simulink model "model"  (R2024a)
settings: Solver=FixedStepAuto  StartTime=0.0  StopTime=100  FixedStep=0.01  RelTol=1e-3
undefined symbols (not defined in the file or in its folder): e0_0, e1_0, e2_0, e3_0, q0, Thrust, vec
libraries: sharedtransform x21, sharedutil x4, aerolibsim3d x2, dspsigops x2, shared6dof x1, sim3dlib x1
(part 2 of 2)

== system model/Quadrotor/Forces in Body frame/Thrust in Inertia Frame ==
  DCM_be : Inport
  Thrust : Inport  Port=2
  Mux : Mux  Inputs=3
  Product1 : Product  Multiplication=Matrix(*)  InputSameDT=on  SaturateOnIntegerOverflow=on  OutDataTypeStr=Inherit: Same as first input
  Reshape : Reshape  OutputDimensionality=Column vector (2-D)
  Transpose : Math  Operator=transpose
  x : Constant  Value=0  SampleTime=-1
  y : Constant  Value=0  SampleTime=-1
  U : Outport
  wires:
  Product1/1 -> U/1
  Mux/1 -> Reshape/1
  y/1 -> Mux/2
  x/1 -> Mux/1
  Reshape/1 -> Product1/2
  Thrust/1 -> Mux/3
  DCM_be/1 -> Transpose/1
  Transpose/1 -> Product1/1

== system model/Quadrotor in body/6DOF NED/Angular Velocity Dyanmics ==
  Moments : Inport  OutDataTypeStr=double
  Bus Creator1 : BusCreator  Inputs=3
  Bus Creator2 : BusCreator  Inputs=3
  Centrifugal Moments : Subsystem
  Demux1 : Demux  Outputs=3
  Demux2 : Demux  Outputs=3
  Inertia Matrix : Constant  Value=InertiaMatrix
  Product2 : Product  Inputs=*/  Multiplication=Matrix(*)  SaturateOnIntegerOverflow=on  OutDataTypeStr=Inherit: Same as first input
  Reshape : Reshape
  Reshape1 : Reshape  OutputDimensionality=Row vector (2-D)
  Sum2 : Sum  Inputs=++|  SaturateOnIntegerOverflow=on
  Wdot Integ : Integrator  InitialCondition=OmegaInitialValues  ContinuousStateAttributes={'p', 'q', 'r'}
  W : Outport
  Wdot : Outport  Port=2  OutDataTypeStr=double  Unit=rad/s^2  VectorParamsAs1DForOutWhenUnconnected=off
  wires:
  Bus Creator2/1 -> Wdot/1  "Wdot"
  Demux2/1 -> Bus Creator2/1  "pdot"
  Demux2/3 -> Bus Creator2/3  "rdot"
  Demux2/2 -> Bus Creator2/2  "qdot"
  Reshape/1 -> Wdot Integ/1, Demux2/1
  Sum2/1 -> Reshape1/1
  Bus Creator1/1 -> Centrifugal Moments/1(w), W/1  "W"
  Demux1/2 -> Bus Creator1/2  "q"
  Demux1/3 -> Bus Creator1/3  "r"
  Wdot Integ/1 -> Demux1/1
  Demux1/1 -> Bus Creator1/1  "p"
  Reshape1/1 -> Product2/1
  Moments/1 -> Sum2/1
  Inertia Matrix/1 -> Product2/2
  Centrifugal Moments/1((I * w) x w) -> Sum2/2
  Product2/1 -> Reshape/1

== system model/Quadrotor in body/6DOF NED/Quaternion Dynamics ==
  w : Inport
  Integrating : Subsystem
  Mux : Mux  Inputs=2
  Quat to Euler : Subsystem
  Quaternions to Direction Cosine Matrix : sharedtransform/Quaternions to  Direction Cosine Matrix  aMode=aMode
  q0_dot : Subsystem
  qvec_dot : Subsystem
  DCM_be : Outport  OutDataTypeStr=double  VectorParamsAs1DForOutWhenUnconnected=off
  Quat : Outport  Port=2  OutDataTypeStr=double  VectorParamsAs1DForOutWhenUnconnected=off
  Euler : Outport  Port=3  OutDataTypeStr=double  VectorParamsAs1DForOutWhenUnconnected=off
  wires:
  Quat to Euler/1(euler) -> Euler/1
  Mux/1 -> Integrating/1(qdot)
  w/1 -> q0_dot/1(w), qvec_dot/1(w)
  Quaternions to Direction Cosine Matrix/1 -> DCM_be/1
  q0_dot/1(q0_dot) -> Mux/1
  qvec_dot/1(qvec_dot) -> Mux/2
  Integrating/1(Quat) -> qvec_dot/2(q), q0_dot/2(q), Quat to Euler/1(q), Quaternions to Direction Cosine Matrix/1, Quat/1

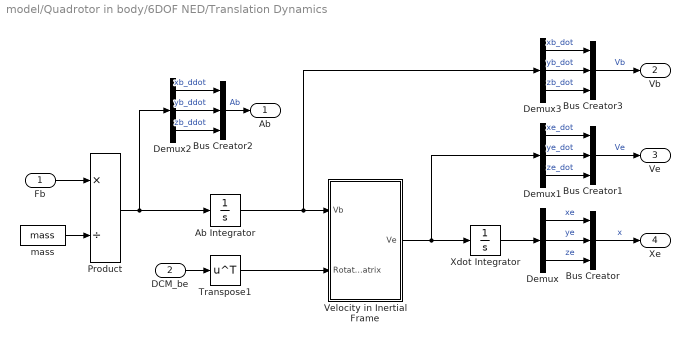
== system model/Quadrotor in body/6DOF NED/Translation Dynamics ==
  Fb : Inport
  DCM_be : Inport  Port=2
  Ab Integrator : Integrator  InitialCondition=VelocityBodyInitialValues  ContinuousStateAttributes={'u', 'v', 'w'}
  Bus Creator{,1..3} (4 alike) : BusCreator  Inputs=3
  Demux{,1..3} (4 alike) : Demux  Outputs=3
  Product : Product  Inputs=*/
  Transpose1 : Math  Operator=transpose  SignedPower=on
  Velocity in Inertial Frame : Subsystem
  Xdot Integrator : Integrator  InitialCondition=PositionReferenceInitialValues  ContinuousStateAttributes={'xr', 'ye', 'ze'}
  mass : Constant  Value=mass
  Ab : Outport  OutDataTypeStr=double  Unit=m/s^2  VectorParamsAs1DForOutWhenUnconnected=off
  Vb : Outport  Port=2  OutDataTypeStr=double  Unit=m/s  VectorParamsAs1DForOutWhenUnconnected=off
  Ve : Outport  Port=3  OutDataTypeStr=double  Unit=m/s  VectorParamsAs1DForOutWhenUnconnected=off
  Xe : Outport  Port=4
  wires:
  Fb/1 -> Product/1
  Product/1 -> Demux2/1, Ab Integrator/1
  Bus Creator3/1 -> Vb/1  "Vb"
  Demux3/2 -> Bus Creator3/2  "yb_dot"
  Demux3/3 -> Bus Creator3/3  "zb_dot"
  Demux3/1 -> Bus Creator3/1  "xb_dot"
  Bus Creator1/1 -> Ve/1  "Ve"
  Demux2/1 -> Bus Creator2/1  "xb_ddot"
  Demux2/2 -> Bus Creator2/2  "yb_ddot"
  Bus Creator2/1 -> Ab/1  "Ab"
  Demux2/3 -> Bus Creator2/3  "zb_ddot"
  Velocity in Inertial Frame/1(Ve) -> Xdot Integrator/1, Demux1/1
  Ab Integrator/1 -> Velocity in Inertial Frame/1(Vb), Demux3/1
  Transpose1/1 -> Velocity in Inertial Frame/2(Rotation Matrix)
  Demux1/1 -> Bus Creator1/1  "xe_dot"
  Demux1/3 -> Bus Creator1/3  "ze_dot"
  Demux/3 -> Bus Creator/3  "ze"
  Xdot Integrator/1 -> Demux/1
  Demux/1 -> Bus Creator/1  "xe"
  Bus Creator/1 -> Xe/1  "x"
  DCM_be/1 -> Transpose1/1
  Demux1/2 -> Bus Creator1/2  "ye_dot"
  Demux/2 -> Bus Creator/2  "ye"
  mass/1 -> Product/2

== system model/Quadrotor in body/Applied Forces in Body frame/Apply Thrust and Gravitational Force ==
  Forces : Inport
  DCM_be : Inport  Port=2
  Forces in Body frame : Subsystem  mask{mass=mass, Gain=9.81}
      mask prompts: Gain "Simulink:blkprm_prompts:GainGain"
      mask TypeOptions Gain:
      | Gravitational Force
      | in Body Frame/g/Gain
      mask DialogControl Gain Prompt: Gain:
  Fb : Outport
  wires:
  Forces/1 -> Forces in Body frame/1(Thrust)
  DCM_be/1 -> Forces in Body frame/2(DCM_be)
  Forces in Body frame/1(Fb) -> Fb/1

== system model/Quadrotor in body/Applied Forces in Body frame/Direct Implementation to Body Forces ==
  Forces : Inport
  DCM_be : Inport  Port=2
  Terminator3 : Terminator
  Fb : Outport
  wires:
  DCM_be/1 -> Terminator3/1
  Forces/1 -> Fb/1

== system model/Quadrotor in body/Forces in Body frame/Gravitational Force in Body Frame ==
  DCM_be : Inport
  Mux : Mux  Inputs=3
  Product1 : Product  Multiplication=Matrix(*)  InputSameDT=on  SaturateOnIntegerOverflow=on  OutDataTypeStr=Inherit: Same as first input
  Reshape : Reshape  OutputDimensionality=Column vector (2-D)
  g : Gain  Gain=Gain
  m : Constant  Value=mass
  x : Constant  Value=0  SampleTime=-1
  y : Constant  Value=0  SampleTime=-1
  FGb : Outport
  wires:
  g/1 -> Mux/3
  DCM_be/1 -> Product1/1
  Reshape/1 -> Product1/2
  m/1 -> g/1
  x/1 -> Mux/1
  y/1 -> Mux/2
  Mux/1 -> Reshape/1
  Product1/1 -> FGb/1

== system model/Quaternion with bit error caculation using quaternion paper/Calculate Omega desired/Skew Matrix ==
  Inport : Inport
  Demux : Demux  Outputs=3
  Matrix Concatenate : Concatenate  NumInputs=3  Mode=Multidimensional array  ConcatenateDimension=2
  Subsystem : Subsystem
  Subsystem1 : Subsystem
  Subsystem2 : Subsystem
  Out1 : Outport
  wires:
  Demux/1 -> Subsystem2/1(Inport), Subsystem1/1(Inport), Subsystem/1(Inport)
  Subsystem1/1(C2) -> Matrix Concatenate/2
  Subsystem2/1(C3) -> Matrix Concatenate/3
  Matrix Concatenate/1 -> Out1/1
  Subsystem/1(C1) -> Matrix Concatenate/1
  Demux/3 -> Subsystem2/3(Inport2), Subsystem1/3(Inport2), Subsystem/3(Inport2)
  Demux/2 -> Subsystem2/2(Inport1), Subsystem1/2(Inport1), Subsystem/2(Inport1)
  Inport/1 -> Demux/1

== system model/Quaternion with bit error caculation using quaternion paper/desired angles dynamcis/To Quaternion Bus ==
  In1 : Inport
  Bus Creator1 : BusCreator  Inputs=q0,vec  OutDataTypeStr=Bus: QuaturnionBus
  Demux2 : Demux
  Mux : Mux  Inputs=3
  q : Outport
  wires:
  Demux2/3 -> Mux/2
  Demux2/1 -> Bus Creator1/1  "q0"
  Demux2/2 -> Mux/1
  Demux2/4 -> Mux/3
  In1/1 -> Demux2/1
  Mux/1 -> Bus Creator1/2  "vec"
  Bus Creator1/1 -> q/1  "q"

== system model/Quaternion with bit error caculation using quaternion paper/desired angles dynamcis/To Quaternion Bus1 ==
  In1 : Inport
  Bus Creator1 : BusCreator  Inputs=q0,vec  OutDataTypeStr=Bus: QuaturnionBus
  Demux2 : Demux
  Mux : Mux  Inputs=3
  q : Outport
  wires:
  Bus Creator1/1 -> q/1  "q"
  Mux/1 -> Bus Creator1/2  "vec"
  In1/1 -> Demux2/1
  Demux2/4 -> Mux/3
  Demux2/2 -> Mux/1
  Demux2/1 -> Bus Creator1/1  "q0"
  Demux2/3 -> Mux/2

== system model/Quaternion with bit error caculation using quaternion paper/desired angles dynamcis/To Quaternion Bus2 ==
  In1 : Inport
  Bus Creator1 : BusCreator  Inputs=q0,vec  OutDataTypeStr=Bus: QuaturnionBus
  Demux2 : Demux
  Mux : Mux  Inputs=3
  q : Outport
  wires:
  Demux2/3 -> Mux/2
  Demux2/1 -> Bus Creator1/1  "q0"
  Demux2/2 -> Mux/1
  Demux2/4 -> Mux/3
  In1/1 -> Demux2/1
  Mux/1 -> Bus Creator1/2  "vec"
  Bus Creator1/1 -> q/1  "q"

== system model/Quaternion with bit error caculation using quaternion paper/desired angles dynamcis/sys1 ==
  u : Inport
  Bus Creator1 : BusCreator  Inputs=3
  Demux1 : Demux  Outputs=3
  State-Space : StateSpace  A=[0 1 0; 0 0 1; -1680 -506 -45]  B=[0; 0; 1680]  C=eye(3)  D=zeros(3,1)  InitialCondition=0
  roll : Outport
  wires:
  State-Space/1 -> Demux1/1
  Demux1/2 -> Bus Creator1/2  "rd_dot"
  Demux1/1 -> Bus Creator1/1  "rd"
  Demux1/3 -> Bus Creator1/3  "rd_ddot"
  u/1 -> State-Space/1
  Bus Creator1/1 -> roll/1

== system model/Quaternion with bit error caculation using quaternion paper/desired angles dynamcis/sys2 ==
  u : Inport
  Bus Creator1 : BusCreator  Inputs=3
  Demux1 : Demux  Outputs=3
  State-Space : StateSpace  A=[0 1 0; 0 0 1; -1680 -506 -45]  B=[0; 0; 1680]  C=eye(3)  D=zeros(3,1)  InitialCondition=0
  pitch : Outport
  wires:
  Bus Creator1/1 -> pitch/1
  u/1 -> State-Space/1
  Demux1/3 -> Bus Creator1/3  "pd_ddot"
  Demux1/1 -> Bus Creator1/1  "pd"
  Demux1/2 -> Bus Creator1/2  "pd_dot"
  State-Space/1 -> Demux1/1

== system model/Quaternion with bit error caculation using quaternion paper/desired angles dynamcis/sys3 ==
  u : Inport
  Bus Creator1 : BusCreator  Inputs=3
  Demux1 : Demux  Outputs=3
  State-Space : StateSpace  A=[0 1 0; 0 0 1; -1680 -506 -45]  B=[0; 0; 1680]  C=eye(3)  D=zeros(3,1)  InitialCondition=0
  yaw : Outport
  wires:
  State-Space/1 -> Demux1/1
  Demux1/2 -> Bus Creator1/2  "yd_dot"
  Demux1/1 -> Bus Creator1/1  "yd"
  Demux1/3 -> Bus Creator1/3  "yd_ddot"
  u/1 -> State-Space/1
  Bus Creator1/1 -> yaw/1

== system model/Quaternion with s  error using quaternion paper/desired angles dynamcis/To Quaternion Bus ==
  In1 : Inport
  Bus Creator1 : BusCreator  Inputs=q0,vec  OutDataTypeStr=Bus: QuaturnionBus
  Demux2 : Demux
  Mux : Mux  Inputs=3
  q : Outport
  wires:
  Demux2/3 -> Mux/2
  Demux2/1 -> Bus Creator1/1  "q0"
  Demux2/2 -> Mux/1
  Demux2/4 -> Mux/3
  In1/1 -> Demux2/1
  Mux/1 -> Bus Creator1/2  "vec"
  Bus Creator1/1 -> q/1  "q"

== system model/Quaternion with s  error using quaternion paper/desired angles dynamcis/To Quaternion Bus1 ==
  In1 : Inport
  Bus Creator1 : BusCreator  Inputs=q0,vec  OutDataTypeStr=Bus: QuaturnionBus
  Demux2 : Demux
  Mux : Mux  Inputs=3
  q : Outport
  wires:
  Bus Creator1/1 -> q/1  "q"
  Mux/1 -> Bus Creator1/2  "vec"
  In1/1 -> Demux2/1
  Demux2/4 -> Mux/3
  Demux2/2 -> Mux/1
  Demux2/1 -> Bus Creator1/1  "q0"
  Demux2/3 -> Mux/2

== system model/Quaternion with s  error using quaternion paper/desired angles dynamcis/To Quaternion Bus2 ==
  In1 : Inport
  Bus Creator1 : BusCreator  Inputs=q0,vec  OutDataTypeStr=Bus: QuaturnionBus
  Demux2 : Demux
  Mux : Mux  Inputs=3
  q : Outport
  wires:
  Demux2/3 -> Mux/2
  Demux2/1 -> Bus Creator1/1  "q0"
  Demux2/2 -> Mux/1
  Demux2/4 -> Mux/3
  In1/1 -> Demux2/1
  Mux/1 -> Bus Creator1/2  "vec"
  Bus Creator1/1 -> q/1  "q"

== system model/Quaternion with s  error using quaternion paper/desired angles dynamcis/sys1 ==
  u : Inport
  Bus Creator1 : BusCreator  Inputs=3
  Demux1 : Demux  Outputs=3
  State-Space : StateSpace  A=[0 1 0; 0 0 1; -1680 -506 -45]  B=[0; 0; 1680]  C=eye(3)  D=zeros(3,1)  InitialCondition=0
  roll : Outport
  wires:
  State-Space/1 -> Demux1/1
  Demux1/2 -> Bus Creator1/2  "rd_dot"
  Demux1/1 -> Bus Creator1/1  "rd"
  Demux1/3 -> Bus Creator1/3  "rd_ddot"
  u/1 -> State-Space/1
  Bus Creator1/1 -> roll/1

== system model/Quaternion with s  error using quaternion paper/desired angles dynamcis/sys2 ==
  u : Inport
  Bus Creator1 : BusCreator  Inputs=3
  Demux1 : Demux  Outputs=3
  State-Space : StateSpace  A=[0 1 0; 0 0 1; -1680 -506 -45]  B=[0; 0; 1680]  C=eye(3)  D=zeros(3,1)  InitialCondition=0
  pitch : Outport
  wires:
  Bus Creator1/1 -> pitch/1
  u/1 -> State-Space/1
  Demux1/3 -> Bus Creator1/3  "pd_ddot"
  Demux1/1 -> Bus Creator1/1  "pd"
  Demux1/2 -> Bus Creator1/2  "pd_dot"
  State-Space/1 -> Demux1/1

== system model/Quaternion with s  error using quaternion paper/desired angles dynamcis/sys3 ==
  u : Inport
  Bus Creator1 : BusCreator  Inputs=3
  Demux1 : Demux  Outputs=3
  State-Space : StateSpace  A=[0 1 0; 0 0 1; -1680 -506 -45]  B=[0; 0; 1680]  C=eye(3)  D=zeros(3,1)  InitialCondition=0
  yaw : Outport
  wires:
  State-Space/1 -> Demux1/1
  Demux1/2 -> Bus Creator1/2  "yd_dot"
  Demux1/1 -> Bus Creator1/1  "yd"
  Demux1/3 -> Bus Creator1/3  "yd_ddot"
  u/1 -> State-Space/1
  Bus Creator1/1 -> yaw/1

== system model/Quaternion with s  error using quaternion paper1/desired angles dynamcis/To Quaternion Bus ==
  In1 : Inport
  Bus Creator1 : BusCreator  Inputs=q0,vec  OutDataTypeStr=Bus: QuaturnionBus
  Demux2 : Demux
  Mux : Mux  Inputs=3
  q : Outport
  wires:
  Demux2/3 -> Mux/2
  Demux2/1 -> Bus Creator1/1  "q0"
  Demux2/2 -> Mux/1
  Demux2/4 -> Mux/3
  In1/1 -> Demux2/1
  Mux/1 -> Bus Creator1/2  "vec"
  Bus Creator1/1 -> q/1  "q"

== system model/Quaternion with s  error using quaternion paper1/desired angles dynamcis/To Quaternion Bus1 ==
  In1 : Inport
  Bus Creator1 : BusCreator  Inputs=q0,vec  OutDataTypeStr=Bus: QuaturnionBus
  Demux2 : Demux
  Mux : Mux  Inputs=3
  q : Outport
  wires:
  Bus Creator1/1 -> q/1  "q"
  Mux/1 -> Bus Creator1/2  "vec"
  In1/1 -> Demux2/1
  Demux2/4 -> Mux/3
  Demux2/2 -> Mux/1
  Demux2/1 -> Bus Creator1/1  "q0"
  Demux2/3 -> Mux/2

== system model/Quaternion with s  error using quaternion paper1/desired angles dynamcis/To Quaternion Bus2 ==
  In1 : Inport
  Bus Creator1 : BusCreator  Inputs=q0,vec  OutDataTypeStr=Bus: QuaturnionBus
  Demux2 : Demux
  Mux : Mux  Inputs=3
  q : Outport
  wires:
  Demux2/3 -> Mux/2
  Demux2/1 -> Bus Creator1/1  "q0"
  Demux2/2 -> Mux/1
  Demux2/4 -> Mux/3
  In1/1 -> Demux2/1
  Mux/1 -> Bus Creator1/2  "vec"
  Bus Creator1/1 -> q/1  "q"

== system model/Quaternion with s  error using quaternion paper1/desired angles dynamcis/sys1 ==
  u : Inport
  Bus Creator1 : BusCreator  Inputs=3
  Demux1 : Demux  Outputs=3
  State-Space : StateSpace  A=[0 1 0; 0 0 1; -1680 -506 -45]  B=[0; 0; 1680]  C=eye(3)  D=zeros(3,1)  InitialCondition=0
  roll : Outport
  wires:
  State-Space/1 -> Demux1/1
  Demux1/2 -> Bus Creator1/2  "rd_dot"
  Demux1/1 -> Bus Creator1/1  "rd"
  Demux1/3 -> Bus Creator1/3  "rd_ddot"
  u/1 -> State-Space/1
  Bus Creator1/1 -> roll/1

== system model/Quaternion with s  error using quaternion paper1/desired angles dynamcis/sys2 ==
  u : Inport
  Bus Creator1 : BusCreator  Inputs=3
  Demux1 : Demux  Outputs=3
  State-Space : StateSpace  A=[0 1 0; 0 0 1; -1680 -506 -45]  B=[0; 0; 1680]  C=eye(3)  D=zeros(3,1)  InitialCondition=0
  pitch : Outport
  wires:
  Bus Creator1/1 -> pitch/1
  u/1 -> State-Space/1
  Demux1/3 -> Bus Creator1/3  "pd_ddot"
  Demux1/1 -> Bus Creator1/1  "pd"
  Demux1/2 -> Bus Creator1/2  "pd_dot"
  State-Space/1 -> Demux1/1

== system model/Quaternion with s  error using quaternion paper1/desired angles dynamcis/sys3 ==
  u : Inport
  Bus Creator1 : BusCreator  Inputs=3
  Demux1 : Demux  Outputs=3
  State-Space : StateSpace  A=[0 1 0; 0 0 1; -1680 -506 -45]  B=[0; 0; 1680]  C=eye(3)  D=zeros(3,1)  InitialCondition=0
  yaw : Outport
  wires:
  State-Space/1 -> Demux1/1
  Demux1/2 -> Bus Creator1/2  "yd_dot"
  Demux1/1 -> Bus Creator1/1  "yd"
  Demux1/3 -> Bus Creator1/3  "yd_ddot"
  u/1 -> State-Space/1
  Bus Creator1/1 -> yaw/1

== system model/Quadrotor/6DOF NED Mixed/Angular Velocity Dyanmics/Centrifugal Moments ==
  w : Inport
  3x3 Cross Product : sharedutil/3x3 Cross Product  aMode=aMode
  Inertia Matrix : Constant  Value=InertiaMatrix
  Product : Product  Multiplication=Matrix(*)  InputSameDT=on  SaturateOnIntegerOverflow=on  OutDataTypeStr=Inherit: Same as first input
  To1D : Reshape
  ToVec : Reshape  OutputDimensionality=Column vector (2-D)
  (I * w) x w : Outport
  wires:
  ToVec/1 -> Product/2
  Product/1 -> To1D/1
  Inertia Matrix/1 -> Product/1
  w/1 -> 3x3 Cross Product/2, ToVec/1
  3x3 Cross Product/1 -> (I * w) x w/1
  To1D/1 -> 3x3 Cross Product/1  "I * w"

== system model/Quadrotor/6DOF NED Mixed/Quaternion Dynamics/Integrating ==
  qdot : Inport
  Initial Euler Angles : Constant  Value=EulerInitialValues
  Quaternion Integration : Integrator  InitialConditionSource=external  InitialCondition=[e0_0 e1_0 e2_0 e3_0]  ContinuousStateAttributes={'q0', 'q1', 'q2', 'q3'}
  Rotation Angles to Quaternions : sharedtransform/Rotation Angles to Quaternions  rotationOrder=ZYX  aMode=aMode
  Selector : Selector  InputPortWidth=3  IndexOptions=Index vector (dialog)  Indices=[3 2 1]  OutputSizes=1
  To Quaternion Bus : Subsystem
  Quat : Outport  OutDataTypeStr=double  VectorParamsAs1DForOutWhenUnconnected=off
  wires:
  Initial Euler Angles/1 -> Selector/1
  Rotation Angles to Quaternions/1 -> Quaternion Integration/2
  Selector/1 -> Rotation Angles to Quaternions/1
  qdot/1 -> Quaternion Integration/1
  Quaternion Integration/1 -> To Quaternion Bus/1(In1)
  To Quaternion Bus/1(q) -> Quat/1

== system model/Quadrotor/6DOF NED Mixed/Quaternion Dynamics/Quat to Euler ==
  q : Inport
  Bus Creator1 : BusCreator  Inputs=3
  Demux : Demux  Outputs=3
  Quaternions to Rotation Angles : sharedtransform/Quaternions to Rotation Angles  rotationOrder=ZYX  aMode=aMode
  Selector : Selector  InputPortWidth=3  IndexOptions=Index vector (dialog)  Indices=[3 2 1]  OutputSizes=1
  Unwrap : dspsigops/Unwrap  tol=pi  InputProcessing=Columns as channels (frame based)  running=off
  euler : Outport
  wires:
  Quaternions to Rotation Angles/1 -> Selector/1
  q/1 -> Quaternions to Rotation Angles/1
  Demux/1 -> Bus Creator1/1  "roll"
  Demux/2 -> Bus Creator1/2  "pitch"
  Selector/1 -> Demux/1
  Bus Creator1/1 -> euler/1  "q_vec"
  Unwrap/1 -> Bus Creator1/3  "yaw"
  Demux/3 -> Unwrap/1  "yaw"

== system model/Quadrotor/6DOF NED Mixed/Quaternion Dynamics/q0_dot ==
  w : Inport  OutDataTypeStr=double
  q : Inport  Port=2
  Bus Selector : BusSelector  OutputSignals=vec  OutputAsBus=on
  Gain : Gain  Gain=-0.5
  Product1 : Product  Inputs=**  Multiplication=Matrix(*)  SaturateOnIntegerOverflow=on  OutDataTypeStr=Inherit: Same as first input
  Reshape2 : Reshape  OutputDimensionality=Column vector (2-D)
  Reshape3 : Reshape  OutputDimensionality=Row vector (2-D)
  q0_dot : Outport
  wires:
  Bus Selector/1 -> Reshape2/1
  Reshape2/1 -> Product1/2
  w/1 -> Reshape3/1
  Reshape3/1 -> Product1/1
  Gain/1 -> q0_dot/1  "q0_dot"
  Product1/1 -> Gain/1  "qvec * w"
  q/1 -> Bus Selector/1

== system model/Quadrotor/6DOF NED Mixed/Quaternion Dynamics/qvec_dot ==
  w : Inport  OutDataTypeStr=double
  q : Inport  Port=2
  3x3 Cross Product : sharedutil/3x3 Cross Product  aMode=aMode
  Add : Sum  Inputs=|++
  Bus Selector1 : BusSelector  OutputSignals=q0
  Bus Selector2 : BusSelector  OutputSignals=vec  OutputAsBus=on
  Gain1 : Gain  Gain=0.5
  Product : Product
  To1D : Reshape
  To1D1 : Reshape
  qvec_dot : Outport
  wires:
  w/1 -> Product/1, To1D1/1  "w"
  Add/1 -> Gain1/1
  Bus Selector1/1 -> Product/2  "<q0>"
  To1D1/1 -> 3x3 Cross Product/2
  q/1 -> Bus Selector1/1, Bus Selector2/1
  To1D/1 -> 3x3 Cross Product/1
  Bus Selector2/1 -> To1D/1
  3x3 Cross Product/1 -> Add/1  "qvec x w"
  Product/1 -> Add/2  "q0.w"
  Gain1/1 -> qvec_dot/1

== system model/Quadrotor/6DOF NED Mixed/Translation Dynamics/Velocity in body Frame ==
  Ve : Inport
  Rotation Matrix : Inport  Port=2
  Product1 : Product  Multiplication=Matrix(*)  InputSameDT=on  SaturateOnIntegerOverflow=on  OutDataTypeStr=Inherit: Same as first input
  Reshape1 : Reshape  OutputDimensionality=Column vector (2-D)
  Reshape2 : Reshape
  Vb : Outport  VectorParamsAs1DForOutWhenUnconnected=off
  wires:
  Ve/1 -> Reshape1/1
  Reshape1/1 -> Product1/2
  Product1/1 -> Reshape2/1
  Reshape2/1 -> Vb/1
  Rotation Matrix/1 -> Product1/1

== system model/Quadrotor/Applied Forces in Body frame/Apply Thrust and Gravitational Force/Forces in Body frame ==
  Thrust : Inport
  DCM_be : Inport  Port=2
  Gravitational Force in Body Frame : Subsystem
  Mux : Mux  Inputs=3
  Reshape : Reshape  OutputDimensionality=Column vector (2-D)
  Reshape2 : Reshape
  Scope12 : Scope
  Sum : Sum  Inputs=|+-
  m : Constant  Value=mass
  x : Constant  Value=0  SampleTime=-1
  y : Constant  Value=0  SampleTime=-1
  Fb : Outport
  wires:
  Gravitational Force in Body Frame/1(FGb) -> Scope12/1, Sum/1
  Sum/1 -> Reshape2/1
  DCM_be/1 -> Gravitational Force in Body Frame/1(DCM_be)
  Thrust/1 -> Mux/3
  Reshape/1 -> Sum/2
  x/1 -> Mux/1
  y/1 -> Mux/2
  Mux/1 -> Reshape/1
  Reshape2/1 -> Fb/1
  m/1 -> Gravitational Force in Body Frame/2(mass)

== system model/Quadrotor in body/6DOF NED/Angular Velocity Dyanmics/Centrifugal Moments ==
  w : Inport
  3x3 Cross Product : sharedutil/3x3 Cross Product  aMode=aMode
  Inertia Matrix : Constant  Value=InertiaMatrix
  Product : Product  Multiplication=Matrix(*)  InputSameDT=on  SaturateOnIntegerOverflow=on  OutDataTypeStr=Inherit: Same as first input
  To1D : Reshape
  ToVec : Reshape  OutputDimensionality=Column vector (2-D)
  (I * w) x w : Outport
  wires:
  To1D/1 -> 3x3 Cross Product/1  "I * w"
  3x3 Cross Product/1 -> (I * w) x w/1
  w/1 -> ToVec/1, 3x3 Cross Product/2
  Inertia Matrix/1 -> Product/1
  Product/1 -> To1D/1
  ToVec/1 -> Product/2

== system model/Quadrotor in body/6DOF NED/Quaternion Dynamics/Integrating ==
  qdot : Inport
  Initial Euler Angles : Constant  Value=EulerInitialValues
  Quaternion Integration : Integrator  InitialConditionSource=external  InitialCondition=[e0_0 e1_0 e2_0 e3_0]  ContinuousStateAttributes={'q0', 'q1', 'q2', 'q3'}
  Rotation Angles to Quaternions : sharedtransform/Rotation Angles to Quaternions  rotationOrder=ZYX  aMode=aMode
  Selector : Selector  InputPortWidth=3  IndexOptions=Index vector (dialog)  Indices=[3 2 1]  OutputSizes=1
  To Quaternion Bus : Subsystem
  Quat : Outport  OutDataTypeStr=double  VectorParamsAs1DForOutWhenUnconnected=off
  wires:
  To Quaternion Bus/1(q) -> Quat/1
  Quaternion Integration/1 -> To Quaternion Bus/1(In1)
  qdot/1 -> Quaternion Integration/1
  Selector/1 -> Rotation Angles to Quaternions/1
  Rotation Angles to Quaternions/1 -> Quaternion Integration/2
  Initial Euler Angles/1 -> Selector/1

== system model/Quadrotor in body/6DOF NED/Quaternion Dynamics/Quat to Euler ==
  q : Inport
  Bus Creator1 : BusCreator  Inputs=3
  Demux : Demux  Outputs=3
  Quaternions to Rotation Angles : sharedtransform/Quaternions to Rotation Angles  rotationOrder=ZYX  aMode=aMode
  Selector : Selector  InputPortWidth=3  IndexOptions=Index vector (dialog)  Indices=[3 2 1]  OutputSizes=1
  Unwrap : dspsigops/Unwrap  tol=pi  InputProcessing=Columns as channels (frame based)  running=off
  euler : Outport
  wires:
  Demux/3 -> Unwrap/1  "yaw"
  Unwrap/1 -> Bus Creator1/3  "yaw"
  Bus Creator1/1 -> euler/1  "q_vec"
  Selector/1 -> Demux/1
  Demux/2 -> Bus Creator1/2  "pitch"
  Demux/1 -> Bus Creator1/1  "roll"
  q/1 -> Quaternions to Rotation Angles/1
  Quaternions to Rotation Angles/1 -> Selector/1

== system model/Quadrotor in body/6DOF NED/Quaternion Dynamics/q0_dot ==
  w : Inport  OutDataTypeStr=double
  q : Inport  Port=2
  Bus Selector : BusSelector  OutputSignals=vec  OutputAsBus=on
  Gain : Gain  Gain=-0.5
  Product1 : Product  Inputs=**  Multiplication=Matrix(*)  SaturateOnIntegerOverflow=on  OutDataTypeStr=Inherit: Same as first input
  Reshape2 : Reshape  OutputDimensionality=Column vector (2-D)
  Reshape3 : Reshape  OutputDimensionality=Row vector (2-D)
  q0_dot : Outport
  wires:
  q/1 -> Bus Selector/1
  Product1/1 -> Gain/1  "qvec * w"
  Gain/1 -> q0_dot/1  "q0_dot"
  Reshape3/1 -> Product1/1
  w/1 -> Reshape3/1
  Reshape2/1 -> Product1/2
  Bus Selector/1 -> Reshape2/1

== system model/Quadrotor in body/6DOF NED/Quaternion Dynamics/qvec_dot ==
  w : Inport  OutDataTypeStr=double
  q : Inport  Port=2
  3x3 Cross Product : sharedutil/3x3 Cross Product  aMode=aMode
  Add : Sum  Inputs=|++
  Bus Selector1 : BusSelector  OutputSignals=q0
  Bus Selector2 : BusSelector  OutputSignals=vec  OutputAsBus=on
  Gain1 : Gain  Gain=0.5
  Product : Product
  To1D : Reshape
  To1D1 : Reshape
  qvec_dot : Outport
  wires:
  Gain1/1 -> qvec_dot/1
  Product/1 -> Add/2  "q0.w"
  3x3 Cross Product/1 -> Add/1  "qvec x w"
  Bus Selector2/1 -> To1D/1
  To1D/1 -> 3x3 Cross Product/1
  q/1 -> Bus Selector2/1, Bus Selector1/1
  To1D1/1 -> 3x3 Cross Product/2
  Bus Selector1/1 -> Product/2  "<q0>"
  Add/1 -> Gain1/1
  w/1 -> To1D1/1, Product/1  "w"

== system model/Quadrotor in body/6DOF NED/Translation Dynamics/Velocity in Inertial Frame ==
  Vb : Inport
  Rotation Matrix : Inport  Port=2
  Product1 : Product  Multiplication=Matrix(*)  InputSameDT=on  SaturateOnIntegerOverflow=on  OutDataTypeStr=Inherit: Same as first input
  Reshape1 : Reshape  OutputDimensionality=Column vector (2-D)
  Reshape2 : Reshape
  Ve : Outport  VectorParamsAs1DForOutWhenUnconnected=off
  wires:
  Reshape2/1 -> Ve/1
  Product1/1 -> Reshape2/1
  Reshape1/1 -> Product1/2
  Vb/1 -> Reshape1/1
  Rotation Matrix/1 -> Product1/1

== system model/Quadrotor in body/Applied Forces in Body frame/Apply Thrust and Gravitational Force/Forces in Body frame ==
  Thrust : Inport
  DCM_be : Inport  Port=2
  Gravitational Force in Body Frame : Subsystem
  Mux : Mux  Inputs=3
  Reshape : Reshape  OutputDimensionality=Column vector (2-D)
  Reshape2 : Reshape
  Scope12 : Scope
  Sum : Sum  Inputs=|+-
  m : Constant  Value=mass
  x : Constant  Value=0  SampleTime=-1
  y : Constant  Value=0  SampleTime=-1
  Fb : Outport
  wires:
  m/1 -> Gravitational Force in Body Frame/2(mass)
  Reshape2/1 -> Fb/1
  Mux/1 -> Reshape/1
  y/1 -> Mux/2
  x/1 -> Mux/1
  Reshape/1 -> Sum/2
  Thrust/1 -> Mux/3
  DCM_be/1 -> Gravitational Force in Body Frame/1(DCM_be)
  Sum/1 -> Reshape2/1
  Gravitational Force in Body Frame/1(FGb) -> Sum/1, Scope12/1

== system model/Quaternion with bit error caculation using quaternion paper/Calculate Omega desired/Skew Matrix/Subsystem ==
  Inport : Inport
  Inport1 : Inport  Port=2
  Inport2 : Inport  Port=3
  Constant3 : Constant  Value=0
  Mux : Mux  Inputs=3
  Terminator : Terminator
  Unary Minus : UnaryMinus
  C1 : Outport
  wires:
  Constant3/1 -> Mux/1
  Unary Minus/1 -> Mux/3
  Inport1/1 -> Unary Minus/1
  Inport2/1 -> Mux/2
  Mux/1 -> C1/1
  Inport/1 -> Terminator/1

== system model/Quaternion with bit error caculation using quaternion paper/Calculate Omega desired/Skew Matrix/Subsystem1 ==
  Inport : Inport
  Inport1 : Inport  Port=2
  Inport2 : Inport  Port=3
  Constant4 : Constant  Value=0
  Mux1 : Mux  Inputs=3
  Terminator : Terminator
  Unary Minus1 : UnaryMinus
  C2 : Outport
  wires:
  Constant4/1 -> Mux1/2
  Inport/1 -> Mux1/3
  Inport2/1 -> Unary Minus1/1
  Unary Minus1/1 -> Mux1/1
  Mux1/1 -> C2/1
  Inport1/1 -> Terminator/1

== system model/Quaternion with bit error caculation using quaternion paper/Calculate Omega desired/Skew Matrix/Subsystem2 ==
  Inport : Inport
  Inport1 : Inport  Port=2
  Inport2 : Inport  Port=3
  Constant5 : Constant  Value=0
  Mux2 : Mux  Inputs=3
  Terminator : Terminator
  Unary Minus2 : UnaryMinus
  C3 : Outport
  wires:
  Inport/1 -> Unary Minus2/1
  Constant5/1 -> Mux2/3
  Mux2/1 -> C3/1
  Unary Minus2/1 -> Mux2/2
  Inport1/1 -> Mux2/1
  Inport2/1 -> Terminator/1

== system model/Quadrotor/6DOF NED Mixed/Quaternion Dynamics/Integrating/To Quaternion Bus ==
  In1 : Inport
  Bus Creator1 : BusCreator  Inputs=q0,vec  OutDataTypeStr=Bus: QuaturnionBus
  Demux2 : Demux
  Mux : Mux  Inputs=3
  q : Outport
  wires:
  Demux2/3 -> Mux/2
  Demux2/1 -> Bus Creator1/1  "q0"
  Demux2/2 -> Mux/1
  Demux2/4 -> Mux/3
  In1/1 -> Demux2/1
  Mux/1 -> Bus Creator1/2  "vec"
  Bus Creator1/1 -> q/1  "q"

== system model/Quadrotor/Applied Forces in Body frame/Apply Thrust and Gravitational Force/Forces in Body frame/Gravitational Force in Body Frame ==
  DCM_be : Inport
  mass : Inport  Port=2
  Mux : Mux  Inputs=3
  Product1 : Product  Multiplication=Matrix(*)  InputSameDT=on  SaturateOnIntegerOverflow=on  OutDataTypeStr=Inherit: Same as first input
  Reshape : Reshape  OutputDimensionality=Column vector (2-D)
  g : Gain  Gain=Gain
  x : Constant  Value=0  SampleTime=-1
  y : Constant  Value=0  SampleTime=-1
  FGb : Outport
  wires:
  Product1/1 -> FGb/1
  Mux/1 -> Reshape/1
  y/1 -> Mux/2
  x/1 -> Mux/1
  g/1 -> Mux/3
  mass/1 -> g/1
  Reshape/1 -> Product1/2
  DCM_be/1 -> Product1/1

== system model/Quadrotor in body/6DOF NED/Quaternion Dynamics/Integrating/To Quaternion Bus ==
  In1 : Inport
  Bus Creator1 : BusCreator  Inputs=q0,vec  OutDataTypeStr=Bus: QuaturnionBus
  Demux2 : Demux
  Mux : Mux  Inputs=3
  q : Outport
  wires:
  Bus Creator1/1 -> q/1  "q"
  Mux/1 -> Bus Creator1/2  "vec"
  In1/1 -> Demux2/1
  Demux2/4 -> Mux/3
  Demux2/2 -> Mux/1
  Demux2/1 -> Bus Creator1/1  "q0"
  Demux2/3 -> Mux/2

== system model/Quadrotor in body/Applied Forces in Body frame/Apply Thrust and Gravitational Force/Forces in Body frame/Gravitational Force in Body Frame ==
  DCM_be : Inport
  mass : Inport  Port=2
  Mux : Mux  Inputs=3
  Product1 : Product  Multiplication=Matrix(*)  InputSameDT=on  SaturateOnIntegerOverflow=on  OutDataTypeStr=Inherit: Same as first input
  Reshape : Reshape  OutputDimensionality=Column vector (2-D)
  g : Gain  Gain=Gain
  x : Constant  Value=0  SampleTime=-1
  y : Constant  Value=0  SampleTime=-1
  FGb : Outport
  wires:
  DCM_be/1 -> Product1/1
  Reshape/1 -> Product1/2
  mass/1 -> g/1
  g/1 -> Mux/3
  x/1 -> Mux/1
  y/1 -> Mux/2
  Mux/1 -> Reshape/1
  Product1/1 -> FGb/1

== matlab function model/Quaternion with s  error using quaternion paper1/MATLAB Function ==
  data: q input Bus: QuaturnionBus size=1; R input size=[3 3]; w input size=[1 3]; qd input Bus: QuaturnionBus size=1; qd_dot input Bus: QuaturnionBus; Rd input size=[3 3]; e output Bus: QuaturnionBus size=1; Re output size=[3 3]; wd output size=[1 3]; we output size=[1 3]; s output
function [e, Re, wd, we, s] = fcn(q, R, w, qd, qd_dot, Rd)

e.q0 = qd.q0 * q.q0 + qd.vec * q.vec';
e.vec = qd.q0 * q.vec - q.q0 * qd.vec + cross(q.vec, qd.vec);
Re = R*Rd';

wd = qd_dot.vec / (qd.q0*eye(3) + Skew(qd.vec));
we = w - wd * Re';
e0_dot = 0.5 * e.vec * we';
evec_dot = 0.5 * (e.q0 * we + cross(e.vec, we));

% parameters
gama1 = 10;
gama2 = 30;
gama3 = 1;
n = 3;
l = 5;
pow = n/l;
eps = 0.01;

de = DeltaE(e.vec, pow ,eps);
s = evec_dot + gama1 * e.vec + gama2 * de + gama3 * we;

function de = DeltaE (e, pow, eps)
    de = e;
    % for i = 1:3
    %     if abs(e(i)) > eps
    %         de(i) = e(i)^pow;
    %     end
    % end
end

function y = Skew(v)
    y = [    0,  -v(3),  v(2);...
          v(3),      0, -v(1);...
         -v(2),   v(1),    0];
end
end

== matlab function model/Quaternion with s  error using quaternion paper/MATLAB Function ==
  data: q input Bus: QuaturnionBus size=1; R input size=[3 3]; w input size=[1 3]; qd input Bus: QuaturnionBus size=1; qd_dot input Bus: QuaturnionBus; Rd input size=[3 3]; e output Bus: QuaturnionBus size=1; Re output size=[3 3]; wd output size=[1 3]; we output size=[1 3]; s output
function [e, Re, wd, we, s] = fcn(q, R, w, qd, qd_dot, Rd)

e.q0 = qd.q0 * q.q0 + qd.vec * q.vec';
e.vec = qd.q0 * q.vec - q.q0 * qd.vec + cross(q.vec, qd.vec);
Re = R*Rd';

wd = qd_dot.vec / (qd.q0*eye(3) + Skew(qd.vec));
we = w - wd * Re';
e0_dot = 0.5 * e.vec * we';
evec_dot = 0.5 * (e.q0 * we + cross(e.vec, we));

% parameters
gama1 = 10;
gama2 = 30;
gama3 = 1;
n = 3;
l = 5;
pow = n/l;
eps = 0.01;

de = DeltaE(e.vec, pow ,eps);
s = evec_dot + gama1 * e.vec + gama2 * de + gama3 * we;

function de = DeltaE (e, pow, eps)
    de = e;
    % for i = 1:3
    %     if abs(e(i)) > eps
    %         de(i) = e(i)^pow;
    %     end
    % end
end

function y = Skew(v)
    y = [    0,  -v(3),  v(2);...
          v(3),      0, -v(1);...
         -v(2),   v(1),    0];
end
end

== matlab function model/Rotation Dynamics Controller/My paper controller/MATLAB Function ==
  data: sr output size=[3 1]; sw output size=[3 1]; wc output size=[3 1]; qw output size=[3 1]; Kr input size=[3 3]; Kw input size=[3 3]; wd_dot output size=[3 1]; R input size=[3 3]; w input size=[3 1]; Rd input size=[3 3]; wd input size=[3 1]
function [sr, sw, wc, qw, wd_dot] = fcn(Kr, Kw, R, w, Rd, wd)

sR = Rd' * R - eye(3);
sr = InvSkew(sR);

wc = Kr * sr;

Tau_w = 16;

wd_dot = Tau_w * (wc-wd);

sw = w - wd;

qw = wd_dot - Kw * sw;

function vec = InvSkew(Mat)
    vec = zeros(3, 1);
    vec(1) = (Mat(3,2) - Mat(2,3)) / 2;
    vec(2) = (Mat(1,3) - Mat(3,1)) / 2;
    vec(3) = (Mat(2,1) - Mat(1,2)) / 2;
end
end

== matlab function model/Translation Dynamics Controller/My paper Translation Controller but for Quaternion/MATLAB Function ==
  data: ep output size=[3 1]; ev output size=[3 1]; s output size=[3 1]; U output size=[3 1]; Fth output size=1; qc_0 output size=1; Kx input size=[3 3]; Kv input size=[3 3]; x input size=[3 1]; v input size=[3 1]; R input size=[3 3]; xd input size=[3 1]; vd input size=[3 1]; ad input size=[3 1]; mass input size=1; qc_vec output size=[1 3]
function [ep, ev, s, U, Fth, qc_0, qc_vec] = fcn(Kx, Kv, x, v, R, xd, vd, ad, mass)

g = 9.81;

ep = x - xd;
ev = v - vd;
s = ev + Kx * ep;
U = ad - Kx * ev - Kv * s;

Ux = U(1);
Uy = U(2);
Uz = U(3);
Mag = 4;
Un = U;
Usat = max(Un,0);


Fth = mass * sqrt(Un(1)^2 + Un(2)^2 + (Un(3) + g)^2);

% qc.q0 = 1; 
% qc.vec = [0,0,0];
q0 = sqrt((mass * (g + Un(3)) / (2 * Fth)) + 1/2);
vec = [-mass * Un(2) / 2 / Fth / q0,...
        mass * Un(1) / 2 / Fth / q0,...
                                    0];
% Fth = mass * (Un(3) + g);
n = sqrt(q0^2+vec(1)^2+vec(2)^2+vec(3)^2);
qc_0 = q0/n;
qc_vec = vec/n;

Fth = mass * (Un(3) + g);

end
